simulink model "PID_TV"  (R2023b)
settings: Solver=FixedStepDiscrete  StartTime=0.0  StopTime=10.0  RelTol=1e-3
model workspace (MAT data in the model file):
  PID_D_param = 0
  PID_I = 1
  PID_I_param = 1
  PID_N = 100
  PID_N_param = 100
  PID_P = Simulink.Signal
  PID_P.DataType = 'double'
  PID_P.Dimensions = -1
  PID_P.DimensionsMode = 'auto'
  PID_P.Complexity = 'auto'
  PID_P.SampleTime = -1
  PID_P.SamplingMode = 'auto'
  PID_P_param = 3
  test = 1
  uh = 1
  wheel_base = Simulink.Parameter
  wheel_base.DataType = 'double'
  wheel_base.Complexity = 'real'
  wheel_base.Dimensions = [0 0]
undefined symbols (not defined in the file): dt, wb
libraries: slpidlib x1
settings Model: ParameterArgumentNames=PID_D_param,PID_I_param,PID_N_param,PID_P_param,test,uh  Creator=ben  LastModifiedBy=ben
settings OptimizationCC: DefaultParameterBehavior=Inlined  EnhancedBackFolding=on  PassReuseOutputArgsAs=Individual arguments  ZeroExternalMemoryAtStartup=off  ZeroInternalMemoryAtStartup=off  OptimizeBlockOrder=speed  DifferentSizesBufferReuse=on  OptimizationCustomize=off  EfficientTunableParamExpr=on
settings DebuggingCC: ParameterTunabilityLossMsg=error
settings SFSimCC: MATLABDynamicMemAlloc=off
settings RTWCC: Description=Embedded Coder  SystemTargetFile=ert.tlc  GenCodeOnly=on  PackageGeneratedCodeAndArtifacts=on  TemplateMakefile=ert_default_tmf  Toolchain=CMake  TargetLang=C++
settings CodeAppCC: ForceParamTrailComments=on  IgnoreCustomStorageClasses=off  OperatorAnnotations=on  SimulinkDataObjDesc=on  SFDataObjDesc=on  InsertBlockDesc=on
settings ERTTargetCC: TargetLangStandard=C++11 (ISO)  GenerateSampleERTMain=on  CodeInterfacePackaging=C++ class  InlinedParameterPlacement=NonHierarchical  RootIOFormat=Structure reference  RTWCAPISignals=on  RTWCAPIParams=on  RTWCAPIRootIO=on  ERTCustomFileTemplate=example_file_process.tlc

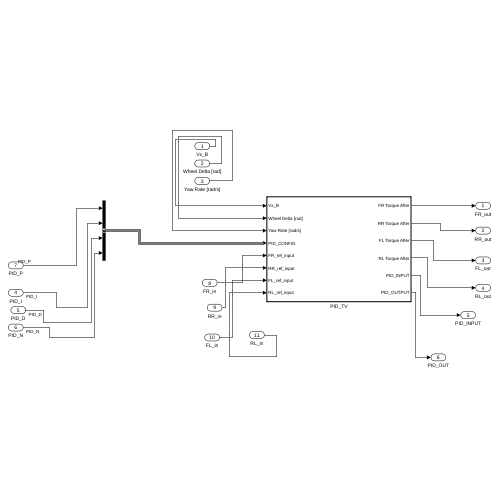
[thumbnail: Simulink's stored preview of the top-level diagram]
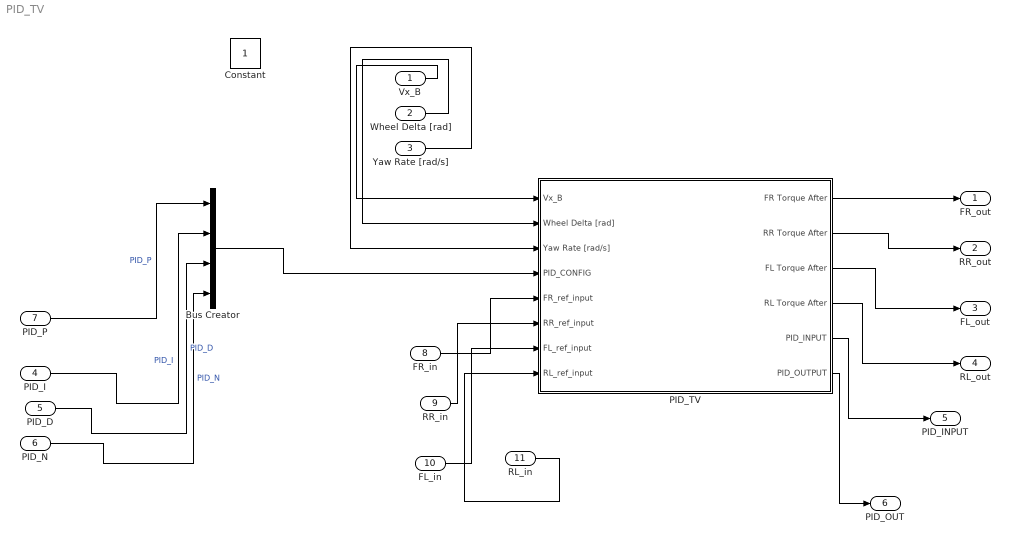
== system PID_TV ==
  Vx_B : Inport
  Wheel Delta [rad] : Inport  Port=2
  Yaw Rate [rad/s] : Inport  Port=3
  PID_I : Inport  Port=4
  PID_D : Inport  Port=5
  PID_N : Inport  Port=6
  PID_P : Inport  Port=7
  FR_in : Inport  Port=8
  RR_in : Inport  Port=9
  FL_in : Inport  Port=10
  RL_in : Inport  Port=11
  Bus Creator : BusCreator  Inputs=4
  PID_TV : Subsystem  TreatAsAtomicUnit=on
  FR_out : Outport
  RR_out : Outport  Port=2
  FL_out : Outport  Port=3
  RL_out : Outport  Port=4
  PID_INPUT : Outport  Port=5
  PID_OUT : Outport  Port=6
  Constant : Constant  IOType=siggen
  wires:
  Vx_B/1 -> PID_TV/1(Vx_B)
  Wheel Delta [rad]/1 -> PID_TV/2(Wheel Delta [rad])
  Yaw Rate [rad/s]/1 -> PID_TV/3(Yaw Rate [rad/s])
  PID_TV/1(FR Torque After) -> FR_out/1
  PID_TV/4(RL Torque After) -> RL_out/1
  PID_TV/3(FL Torque After) -> FL_out/1
  PID_TV/2(RR Torque After) -> RR_out/1
  PID_P/1 -> Bus Creator/1  "PID_P"
  PID_I/1 -> Bus Creator/2  "PID_I"
  PID_D/1 -> Bus Creator/3  "PID_D"
  PID_N/1 -> Bus Creator/4  "PID_N"
  Bus Creator/1 -> PID_TV/4(PID_CONFIG)
  FR_in/1 -> PID_TV/5(FR_ref_input)
  RR_in/1 -> PID_TV/6(RR_ref_input)
  FL_in/1 -> PID_TV/7(FL_ref_input)
  RL_in/1 -> PID_TV/8(RL_ref_input)
  PID_TV/5(PID_INPUT) -> PID_INPUT/1
  PID_TV/6(PID_OUTPUT) -> PID_OUT/1

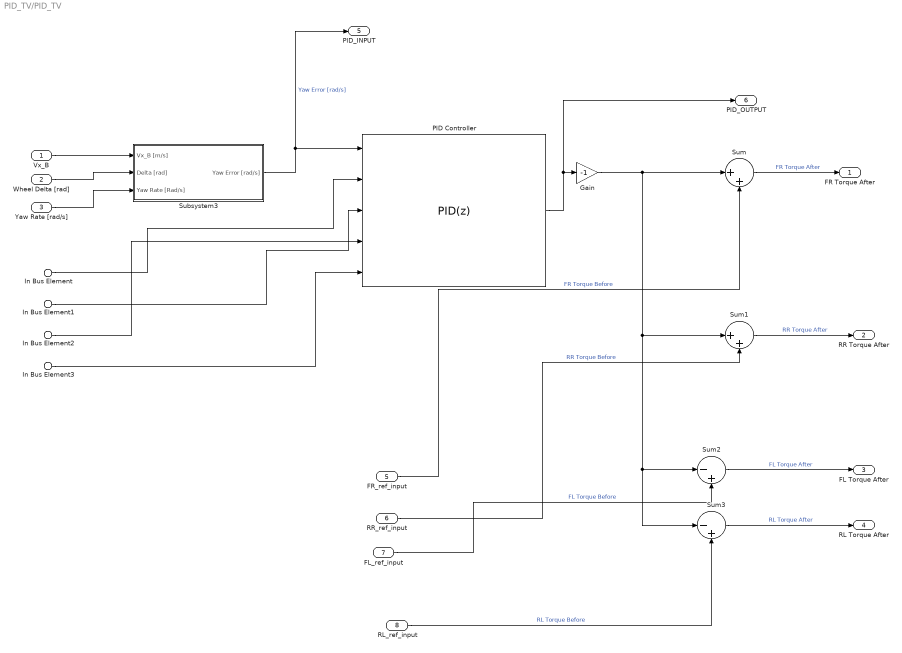
== system PID_TV/PID_TV ==
  Vx_B : Inport
  Wheel Delta [rad] : Inport  Port=2
  Yaw Rate [rad/s] : Inport  Port=3
  In Bus Element : Inport  Port=4  PortName=PID_CONFIG  Element=PID_P
  In Bus Element1 : Inport  Port=4  PortName=PID_CONFIG  Element=PID_I
  In Bus Element2 : Inport  Port=4  PortName=PID_CONFIG  Element=PID_D
  In Bus Element3 : Inport  Port=4  PortName=PID_CONFIG  Element=PID_N
  FR_ref_input : Inport  Port=5
  RR_ref_input : Inport  Port=6
  FL_ref_input : Inport  Port=7
  RL_ref_input : Inport  Port=8
  Gain : Gain  Gain=-1
  PID Controller : slpidlib/PID Controller  Controller=PID  Form=Parallel  TimeDomain=Discrete-time  UseExternalTs=off  SampleTime=dt  IntegratorMethod=Forward Euler  FilterMethod=Forward Euler  ControllerParametersSource=external  P=1  I=1  UseKiTs=off  D=0  N=100  UseFilter=on  TunerSelectOption=Transfer Function Based (PID Tuner App)  InitialConditionSource=internal  InitialConditionForIntegrator=0  InitialConditionForFilter=0  DifferentiatorICPrevScaledInput=0  ExternalReset=none  TrackingMode=off  Kt=1  LimitOutput=off  SatLimitsSource=internal  UpperSaturationLimit=inf  LowerSaturationLimit=-inf  LinearizeAsGain=on  AntiWindupMode=none  Kb=1  LimitIntegrator=off  UpperIntegratorSaturationLimit=inf  LowerIntegratorSaturationLimit=-inf  POutMin=[]  POutMax=[]  IOutMin=[]  IOutMax=[]  DOutMin=[]  DOutMax=[]  NOutMin=[]  NOutMax=[]  SumOutMin=[]  SumOutMax=[]  SaturationOutMin=[]  SaturationOutMax=[]  PParamMin=[]  PParamMax=[]  IParamMin=[]  IParamMax=[]  DParamMin=[]  DParamMax=[]  NParamMin=[]  NParamMax=[]  KbParamMin=[]  KbParamMax=[]  KtParamMin=[]  KtParamMax=[]  KbOutMin=[]  KbOutMax=[]  KtOutMin=[]  KtOutMax=[]  IntegratorOutMin=[]  IntegratorOutMax=[]  FilterOutMin=[]  FilterOutMax=[]  SumI1OutMin=[]  SumI1OutMax=[]  SumI2OutMin=[]  SumI2OutMax=[]  SumI3OutMin=[]  SumI3OutMax=[]  SumI4OutMin=[]  SumI4OutMax=[]  SumDOutMin=[]  SumDOutMax=[]  DifferentiatorOutMin=[]  DifferentiatorOutMax=[]  FilterDiffOutCoefMin=[]  FilterDiffOutCoefMax=[]  ReciprocalOutMin=[]  ReciprocalOutMax=[]  SumDenOutMin=[]  SumDenOutMax=[]  SumNumOutMin=[]  SumNumOutMax=[]  DivideOutMin=[]  DivideOutMax=[]  UdiffTsProdOutMin=[]  UdiffTsProdOutMax=[]  NTsProdOutMin=[]  NTsProdOutMax=[]  UintegralTsProdOutMin=[]  UintegralTsProdOutMax=[]  UngainTsProdOutMin=[]  UngainTsProdOutMax=[]  ClampingZeroOutDataTypeStr=Inherit: Inherit via back propagation  ClampingZeroOutMin=[]  ClampingZeroOutMax=[]  FilterDenConstantOutDataTypeStr=Inherit: Inherit via back propagation  FilterDenConstantOutMin=[]  FilterDenConstantOutMax=[]  PCopyOutDataTypeStr=Inherit: Inherit via back propagation  PCopyOutMin=[]  PCopyOutMax=[]  NCopyOutDataTypeStr=Inherit: Inherit via back propagation  NCopyOutMin=[]  NCopyOutMax=[]  IntegratorContinuousStateAttributes=''  IntegratorStateMustResolveToSignalObject=off  IntegratorRTWStateStorageClass=Auto  FilterContinuousStateAttributes=''  FilterStateMustResolveToSignalObject=off  FilterRTWStateStorageClass=Auto  ParallelPVariant=ExternalParameters  IdealPVariant=Disabled  IVariant=ExternalParameters  DVariant=ExternalParameters  IntegratorVariant=Discrete  SatVariant=Disabled  AWVariant=Passthrough  PCopyVariant=Disabled  TRVariant=Disabled  FdbkBlocksVariant=Forward  IdealPFdbkVariant=Disabled  SatFdbkVariant=Disabled  DerivativeFilterVariant=ForwardEulerFilter  NVariant=ExternalParameters  NCopyVariant=Disabled  FilterICVariant=InternalICsFilter  IntegratorICVariant=InternalICs  ExternalResetVariant=Disabled  TRSumVariant=Passthrough  SumFdbkVariant=Disabled  SumVariant=Sum_PID  TsampFilterVariant=InternalTs  TsampNgainVariant=Passthrough  TsampIntegralVariant=Disabled_SignalSpec  ExternalSaturationOutDataTypeStr=Inherit: Same as second input
  Subsystem3 : Subsystem
  Sum : Sum  Inputs=|++
  Sum1 : Sum  Inputs=|++
  Sum2 : Sum  Inputs=|-+
  Sum3 : Sum  Inputs=|-+
  FR Torque After : Outport
  RR Torque After : Outport  Port=2
  FL Torque After : Outport  Port=3
  RL Torque After : Outport  Port=4
  PID_INPUT : Outport  Port=5
  PID_OUTPUT : Outport  Port=6
  wires:
  Sum2/1 -> FL Torque After/1  "FL Torque After"
  Sum3/1 -> RL Torque After/1  "RL Torque After"
  FL_ref_input/1 -> Sum2/2  "FL Torque Before"
  Sum/1 -> FR Torque After/1  "FR Torque After"
  Sum1/1 -> RR Torque After/1  "RR Torque After"
  RL_ref_input/1 -> Sum3/2  "RL Torque Before"
  Subsystem3/1(Yaw Error [rad/s]) -> PID_INPUT/1, PID Controller/1  "Yaw Error [rad/s]"
  FR_ref_input/1 -> Sum/2  "FR Torque Before"
  Gain/1 -> Sum/1, Sum3/1, Sum2/1, Sum1/1
  RR_ref_input/1 -> Sum1/2  "RR Torque Before"
  PID Controller/1 -> PID_OUTPUT/1, Gain/1
  Vx_B/1 -> Subsystem3/1(Vx_B [m/s])
  Wheel Delta [rad]/1 -> Subsystem3/2(Delta [rad])
  Yaw Rate [rad/s]/1 -> Subsystem3/3(Yaw Rate [Rad/s])
  In Bus Element3/1 -> PID Controller/5
  In Bus Element1/1 -> PID Controller/3
  In Bus Element2/1 -> PID Controller/4
  In Bus Element/1 -> PID Controller/2

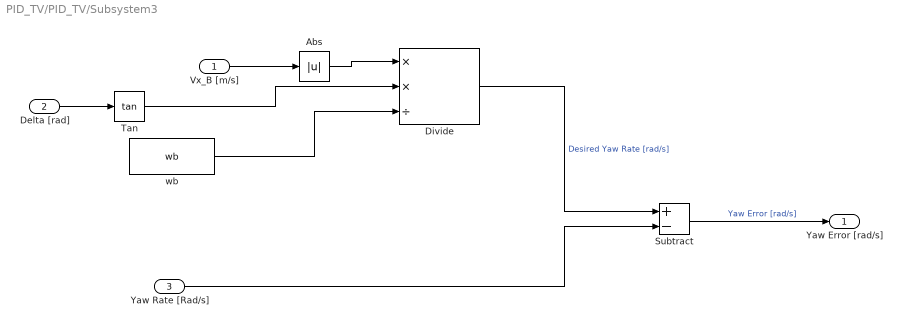
== system PID_TV/PID_TV/Subsystem3 ==
  Vx_B [m/s] : Inport
  Delta [rad] : Inport  Port=2
  Yaw Rate [Rad/s] : Inport  Port=3
  Abs : Abs  SaturateOnIntegerOverflow=off
  Divide : Product  Inputs=**/
  Subtract : Sum  Inputs=+-
  Tan : Trigonometry  Operator=tan
  wb : Constant  Value=wb  OutMin=[0]  OutMax=[10000]
  Yaw Error [rad/s] : Outport
  wires:
  Tan/1 -> Divide/2
  Delta [rad]/1 -> Tan/1
  wb/1 -> Divide/3
  Subtract/1 -> Yaw Error [rad/s]/1  "Yaw Error [rad/s]"
  Yaw Rate [Rad/s]/1 -> Subtract/2
  Divide/1 -> Subtract/1  "Desired Yaw Rate [rad/s]"
  Abs/1 -> Divide/1
  Vx_B [m/s]/1 -> Abs/1
